simulink subsystem "PieroCV"  (R2022b)
settings: Solver=VariableStepAuto  StartTime=0.0  StopTime=10.0  RelTol=1e-3
settings Model: Creator=David  LastModifiedBy=Usuario

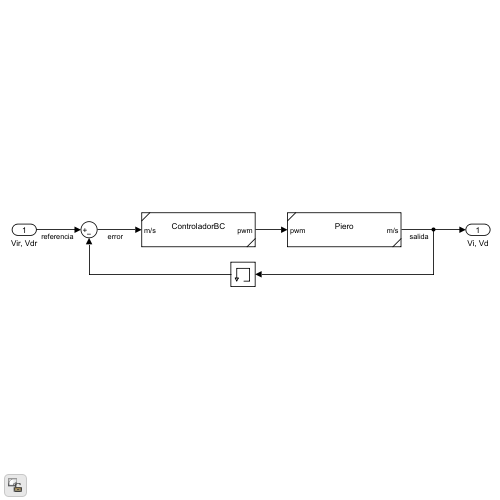
[thumbnail: Simulink's stored preview of the top-level diagram]
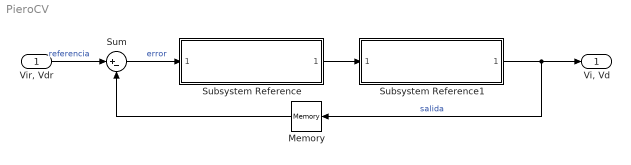
== system PieroCV ==
  "Vir, Vdr" : Inport
  Memory : Memory
  Subsystem Reference : Subsystem  ReferencedSubsystem=ControladorBC
  Subsystem Reference1 : Subsystem  ReferencedSubsystem=Piero
  Sum : Sum  Inputs=|+-
  "Vi, Vd" : Outport
  wires:
  Subsystem Reference1/1 -> "Vi, Vd"/1, Memory/1  "salida"
  Sum/1 -> Subsystem Reference/1  "error"
  Memory/1 -> Sum/2
  "Vir, Vdr"/1 -> Sum/1  "referencia"
  Subsystem Reference/1 -> Subsystem Reference1/1
